simulink model "Decoder_8_4"  (R2017a)
settings: Solver=ode45  StartTime=0.0  StopTime=1e-3  RelTol=1e-3  EnableMultiTasking=on
settings Model: Creator=robertoeduardo  LastModifiedBy=Jesus
settings DataIOCC: LimitDataPoints=on  SaveFormat=Array
settings OptimizationCC: LifeSpan=inf
settings DebuggingCC: UnderspecifiedInitializationDetection=Classic  MergeDetectMultiDrivingBlocksExec=none  SolverPrmCheckMsg=warning  SFUnexpectedBacktrackingDiag=warning  SFNoUnconditionalDefaultTransitionDiag=warning  SFExecutionAtInitializationDiag=none
settings HardwareCC: ProdBitPerPointer=32  ProdBitPerSizeT=32  ProdBitPerPtrDiffT=32  ProdLargestAtomicFloat=None  ProdIntDivRoundTo=Undefined  ProdEndianess=Unspecified  ProdWordSize=32  ProdHWDeviceType=32-bit Generic
settings ModelReferenceCC: PropagateSignalLabelsOutOfModel=off
settings GRTTargetCC: TargetLangStandard=C89/C90 (ANSI)  GeneratePreprocessorConditionals=Disable all
settings ConfigComp: CovMetricSettings=dw  CovHtmlReporting=on  CovSaveCumulativeToWorkspaceVar=on  CovSaveSingleToWorkspaceVar=on  CovExternalEMLEnable=off

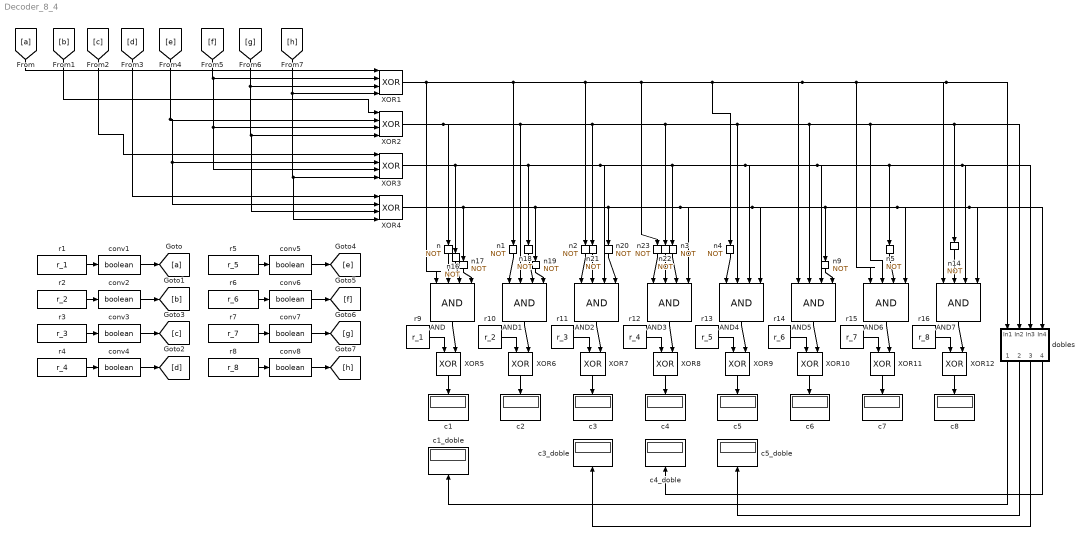
== system Decoder_8_4 ==
  AND{,1..7} (8 alike) : Logic  Inputs=4  IconShape=distinctive  AllPortsSameDT=off  OutDataTypeStr=boolean
  XOR{1..4} (4 alike) : Logic  Operator=XOR  Inputs=4  IconShape=distinctive  AllPortsSameDT=off  OutDataTypeStr=boolean
  XOR{5..12} (8 alike) : Logic  Operator=XOR  IconShape=distinctive  AllPortsSameDT=off  OutDataTypeStr=boolean
  c{1..8} (8 alike) : Display
  c1_doble : Display
  c3_doble : Display
  c4_doble : Display
  c5_doble : Display
  conv{1..8} (8 alike) : DataTypeConversion  OutDataTypeStr=boolean
  dobles : Subsystem
  n{,1..5,9,14,16..23} (16 alike) : Logic  Operator=NOT  Inputs=4  IconShape=distinctive  AllPortsSameDT=off  OutDataTypeStr=boolean
  r1 : FromWorkspace  VariableName=r_1  SampleTime=0
  r10 : FromWorkspace  VariableName=r_2  SampleTime=0
  r11 : FromWorkspace  VariableName=r_3  SampleTime=0
  r12 : FromWorkspace  VariableName=r_4  SampleTime=0
  r13 : FromWorkspace  VariableName=r_5  SampleTime=0
  r14 : FromWorkspace  VariableName=r_6  SampleTime=0
  r15 : FromWorkspace  VariableName=r_7  SampleTime=0
  r16 : FromWorkspace  VariableName=r_8  SampleTime=0
  r2 : FromWorkspace  VariableName=r_2  SampleTime=0
  r3 : FromWorkspace  VariableName=r_3  SampleTime=0
  r4 : FromWorkspace  VariableName=r_4  SampleTime=0
  r5 : FromWorkspace  VariableName=r_5  SampleTime=0
  r6 : FromWorkspace  VariableName=r_6  SampleTime=0
  r7 : FromWorkspace  VariableName=r_7  SampleTime=0
  r8 : FromWorkspace  VariableName=r_8  SampleTime=0
  r9 : FromWorkspace  VariableName=r_1  SampleTime=0
  wires:
  r2/1 -> conv2/1
  r3/1 -> conv3/1
  r4/1 -> conv4/1
  r5/1 -> conv5/1
  r1/1 -> conv1/1
  r6/1 -> conv6/1
  r7/1 -> conv7/1
  r8/1 -> conv8/1
  n9/1 -> AND5/4
  n14/1 -> AND7/2
  AND/1 -> XOR5/2
  AND1/1 -> XOR6/2
  AND2/1 -> XOR7/2
  AND3/1 -> XOR8/2
  AND4/1 -> XOR9/2
  AND5/1 -> XOR10/2
  AND6/1 -> XOR11/2
  AND7/1 -> XOR12/2
  r9/1 -> XOR5/1
  r10/1 -> XOR6/1
  r11/1 -> XOR7/1
  r12/1 -> XOR8/1
  r13/1 -> XOR9/1
  r14/1 -> XOR10/1
  r15/1 -> XOR11/1
  r16/1 -> XOR12/1
  XOR5/1 -> c1/1
  XOR6/1 -> c2/1
  XOR7/1 -> c3/1
  XOR8/1 -> c4/1
  XOR9/1 -> c5/1
  XOR10/1 -> c6/1
  XOR11/1 -> c7/1
  XOR12/1 -> c8/1
  conv1/1 -> [a]
  conv4/1 -> [d]
  conv2/1 -> [b]
  conv3/1 -> [c]
  conv5/1 -> [e]
  conv6/1 -> [f]
  conv7/1 -> [g]
  conv8/1 -> [h]
  [a] -> XOR1/1
  [b] -> XOR2/1
  [c] -> XOR3/1
  [f] -> XOR3/3, XOR2/3, XOR1/2
  [g] -> XOR1/3, XOR4/3, XOR2/4
  [h] -> XOR1/4, XOR4/4, XOR3/4
  XOR1/1 -> AND/1, n1/1, n2/1, n23/1, n4/1, AND5/1, AND6/1, AND7/1, dobles/1(In1)
  XOR4/1 -> n17/1, n20/1, AND3/4, AND4/4, n9/1, dobles/4(In4), AND7/4, AND6/4, n19/1
  XOR2/1 -> n/1, AND1/2, n21/1, n22/1, AND4/2, AND6/2, dobles/2(In2), n14/1, AND5/2
  XOR3/1 -> n16/1, AND2/3, AND4/3, n5/1, AND7/3, dobles/3(In3), AND5/3, n3/1, n18/1
  dobles/1(Out1) -> c1_doble/1
  dobles/2(Out2) -> c5_doble/1
  dobles/3(Out3) -> c3_doble/1
  dobles/4(Out4) -> c4_doble/1
  [e] -> XOR4/2, XOR3/2, XOR2/2
  [d] -> XOR4/1
  n/1 -> AND/2
  n16/1 -> AND/3
  n17/1 -> AND/4
  n1/1 -> AND1/1
  n18/1 -> AND1/3
  n19/1 -> AND1/4
  n2/1 -> AND2/1
  n20/1 -> AND2/4
  n21/1 -> AND2/2
  n3/1 -> AND3/3
  n22/1 -> AND3/2
  n23/1 -> AND3/1
  n4/1 -> AND4/1
  n5/1 -> AND6/3

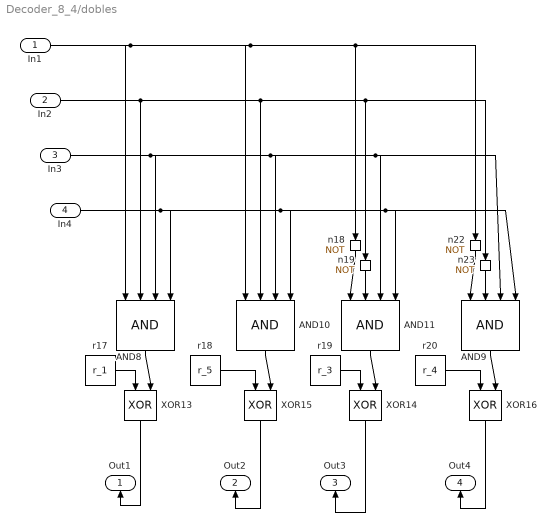
== system Decoder_8_4/dobles ==
  In1 : Inport
  In2 : Inport  Port=2
  In3 : Inport  Port=3
  In4 : Inport  Port=4
  AND{8..11} (4 alike) : Logic  Inputs=4  IconShape=distinctive  AllPortsSameDT=off  OutDataTypeStr=boolean
  XOR{13..16} (4 alike) : Logic  Operator=XOR  IconShape=distinctive  AllPortsSameDT=off  OutDataTypeStr=boolean
  n{18..19,22..23} (4 alike) : Logic  Operator=NOT  Inputs=4  IconShape=distinctive  AllPortsSameDT=off  OutDataTypeStr=boolean
  r17 : FromWorkspace  VariableName=r_1  SampleTime=0
  r18 : FromWorkspace  VariableName=r_5  SampleTime=0
  r19 : FromWorkspace  VariableName=r_3  SampleTime=0
  r20 : FromWorkspace  VariableName=r_4  SampleTime=0
  Out1 : Outport
  Out2 : Outport  Port=2
  Out3 : Outport  Port=3
  Out4 : Outport  Port=4
  wires:
  XOR14/1 -> Out3/1
  XOR15/1 -> Out2/1
  XOR13/1 -> Out1/1
  r17/1 -> XOR13/1
  n23/1 -> AND9/2
  r19/1 -> XOR14/1
  n22/1 -> AND9/1
  AND8/1 -> XOR13/2
  r20/1 -> XOR16/1
  AND10/1 -> XOR15/2
  r18/1 -> XOR15/1
  n19/1 -> AND11/2
  n18/1 -> AND11/1
  AND11/1 -> XOR14/2
  AND9/1 -> XOR16/2
  XOR16/1 -> Out4/1
  In1/1 -> AND8/1, AND10/1, n18/1, n22/1
  In4/1 -> AND8/4, AND10/4, AND11/4, AND9/4
  In2/1 -> AND8/2, AND10/2, n19/1, n23/1
  In3/1 -> AND8/3, AND10/3, AND11/3, AND9/3
